simulink model "hw_sodim"  (R2017b)
settings: Solver=VariableStepAuto  StartTime=0.0  StopTime=inf  RelTol=1e-3  EnableMultiTasking=on
undefined symbols (not defined in the file or in its folder): A, N
libraries: xbsIndex_r4 x1, JTAGRuntimeCosim_r4 x1
settings Model: Creator=szekelyi  LastModifiedBy=kovacs.attila
settings DataIOCC: LimitDataPoints=on
settings OptimizationCC: LifeSpan=inf
settings DebuggingCC: AllowSymbolicDim=off  SFUnexpectedBacktrackingDiag=warning  SFNoUnconditionalDefaultTransitionDiag=warning  SFExecutionAtInitializationDiag=none
settings ModelReferenceCC: PropagateSignalLabelsOutOfModel=off
settings CodeAppCC: StateflowObjectComments=on
settings GRTTargetCC: TargetLangStandard=C89/C90 (ANSI)
settings ConfigComp: CovMetricSettings=dw  CovHtmlReporting=on  CovSaveCumulativeToWorkspaceVar=on  CovSaveSingleToWorkspaceVar=on  CovExternalEMLEnable=off

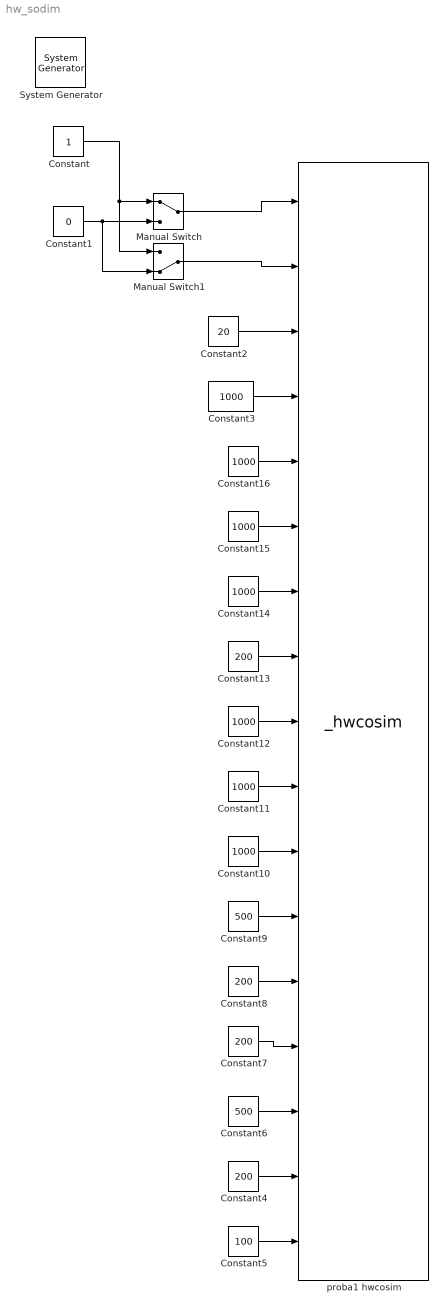
== system hw_sodim ==
  " System Generator" : xbsIndex_r4/ System Generator  Tag=genX  xilinxfamily=artix7  part=xc7a200t  speed=-2  package=fbg676  synthesis_tool=Vivado  clock_wrapper=Clock Enables  directory=./netlist  proj_type=Vivado  Synth_file=Vivado Synthesis Defaults  Impl_file=Vivado Implementation Defaults  testbench=off  simulink_period=1  sysclk_period=10  dcm_input_clock_period=10  incr_netlist=off  trim_vbits=Everywhere in SubSystem  dbl_ovrd=According to Block Masks  core_generation=According to Block Masks  run_coregen=off  deprecated_control=off  eval_field=0  block_type=sysgen
  Constant : Constant
  Constant1 : Constant  Value=0
  Constant{3,10..12,14..16} (7 alike) : Constant  Value=1000
  Constant{4,7..8,13} (4 alike) : Constant  Value=200
  Constant2 : Constant  Value=20
  Constant5 : Constant  Value=100
  Constant6 : Constant  Value=500
  Constant9 : Constant  Value=500
  Manual Switch : ManualSwitch
  Manual Switch1 : ManualSwitch  CurrentSetting=0
  proba1 hwcosim : JTAGRuntimeCosim_r4/_hwcosim  clkSrc=Single Stepped  hasCombinationalPath=on  bitfileName=D:\Diak\Kovacs_Attila\Demo\netlist\proba1.bit  skipConfig=off  dispPartInfo=off  useZynqReconfigScript=on  cable=Auto Detect  speed=N/A  cablePort=N/A  cableLocation=Local  shareCable=off  design_xtable=|  engineDll=JTAGCosimEngine.dll  cableWaitTime=10  bscanPos=-1  IRLengths=[]  useWaitBox=1  hasBufgmux=on  Scheme=Cosim  useCmdProc=1  hasProc=0  useImpact=0  printLogFile=0  userChain=2  block_type=jtagcosim
      | {
      |     'clkWrapper' => 'proba1',
      |     'burstMode' => false,
      |     'burstFifoDepth' => '1024',
      |     'shared_memories' => {},
      |     'clocksGcd' => 1,
      |     'device' => {
      |       'family' => 'artix7',
      |       'part' => 'xc7a35t',
      |       'package' => 'cpg236',
      |       'speed' => '-1',
      |     },
      |     'ports' => {
      |       'start' => {
      |         'direction' => 'in',
      |         'width' => 1,
      |         'name' => 'start',
      |         'period' => 1,
      |         'icon_text' => 'start',
      |         'type' => 'Bool',
      |         'arithmetic_type' => 'xlUnsigned',
      |         'dat_file' => 'proba1_jtag_domain_start.dat',
      |         'bin_pt' => 0,
      |         'addr_offset' => 0,
      |         'bd_port_index' => 0,
      |       },
      |       'reset' => {
      |         'direction' => 'in',
      |         'width' => 1,
      |         'name' => 'reset',
      |         'period' => 1,
      |         'icon_text' => 'reset',
      |         'type' => 'Bool',
      |         'arithmetic_type' => 'xlUnsigned',
      |         'dat_file' => 'proba1_jtag_domain_reset.dat',
      |         'bin_pt' => 0,
      |         'addr_offset' => 4,
      |         'bd_port_index' => 1,
      |       },
      |       'minval' => {
      |         'direction' => 'in',
      |         'width' => 32,
      |         'name' => 'minval',
      |         'period' => 1,
      |         'icon_text' => 'minval',
      |         'type' => 'UFix_32_0',
      |         'arithmetic_type' => 'xlUnsigned',
      |         'dat_file' => 'proba1_jtag_domain_minval.dat',
      |         'bin_pt' => 0,
      |         'addr_offset' => 8,
      |         'bd_port_index' => 2,
      |       },
      |       'maxval' => {
      |         'direction' => 'in',
      |         'width' => 32,
      |         'name' => 'maxval',
      |         'period' => 1,
      |         'icon_text' => 'maxval',
      |         'type' => 'UFix_32_0',
      |         'arithmetic_type' => 'xlUnsigned',
      |         'dat_file' => 'proba1_jtag_domain_maxval.dat',
      |         'bin_pt' => 0,
      |         'addr_offset' => 12,
      |         'bd_port_index' => 3,
      |       },
      |       'h9' => {
      |         'direction' => 'in',
      |         'width' => 32,
      |         'name' => 'h9',
      |         'period' => 1,
      |         'icon_text' => 'h9',
      |         'type' => 'UFix_32_0',
      |         'arithmetic_type' => 'xlUnsigned',
      |         'dat_file' => 'proba1_jtag_domain_h9.dat',
      |         'bin_pt' => 0,
      |         'addr_offset' => 16,
      |         'bd_port_index' => 4,
      |       },
      |       'h8' => {
      |         'direction' => 'in',
      |         'width' => 32,
      |         'name' => 'h8',
      |         'period' => 1,
      |         'icon_text' => 'h8',
      |         'type' => 'UFix_32_0',
      |         'arithmetic_type' => 'xlUnsigned',
      |         'dat_file' => 'proba1_jtag_domain_h8.dat',
      |         'bin_pt' => 0,
      |         'addr_offset' => 20,
      |         'bd_port_index' => 5,
      |       },
      |       'h7' => {
      |         'direction' => 'in',
      |         'width' => 32,
      |         'name' => 'h7',
      |         'period' => 1,
      |         'icon_text' => 'h7',
      |         'type' => 'UFix_32_0',
      |         'arithmetic_type' => 'xlUnsigned',
      |         'dat_file' => 'proba1_jtag_domain_h7.dat',
      |         'bin_pt' => 0,
      |         'addr_offset' => 24,
      |         'bd_port_index' => 6,
      |       },
      |       'h6' => {
      |         'direction' => 'in',
      |         'width' => 32,
      |         'name' => 'h6',
      |         'period' => 1,
      |         'icon_text' => 'h6',
      |         'type' => 'UFix_32_0',
      |         'arithmetic_type' => 'xlUnsigned',
      |         'dat_file' => 'proba1_jtag_domain_h6.dat',
      |         'bin_pt' => 0,
      |         'addr_offset' => 28,
      |         'bd_port_index' => 7,
      |       },
      |       'h5' => {
      |         'direction' => 'in',
      |         'width' => 32,
      |         'name' => 'h5',
      |         'period' => 1,
      |         'icon_text' => 'h5',
      |         'type' => 'UFix_32_0',
      |         'arithmetic_type' => 'xlUnsigned',
      |         'dat_file' => 'proba1_jtag_domain_h5.dat',
      |         'bin_pt' => 0,
      |         'addr_offset' => 32,
      |         'bd_port_index' => 8,
      |       },
      |       'h4' => {
      |         'direction' => 'in',
      |         'width' => 32,
      |         'name' => 'h4',
      |         'period' => 1,
      |         'icon_text' => 'h4',
      |         'type' => 'UFix_32_0',
      |         'arithmetic_type' => 'xlUnsigned',
      |         'dat_file' => 'proba1_jtag_domain_h4.dat',
      |         'bin_pt' => 0,
      |         'addr_offset' => 36,
      |         'bd_port_index' => 9,
      |       },
      |       'h3' => {
      |         'direction' => 'in',
      |         'width' => 32,
      |         'name' => 'h3',
      |         'period' => 1,
      |         'icon_text' => 'h3',
      |         'type' => 'UFix_32_0',
      |         'arithmetic_type' => 'xlUnsigned',
      |         'dat_file' => 'proba1_jtag_domain_h3.dat',
      |         'bin_pt' => 0,
      |         'addr_offset' => 40,
      |         'bd_port_index' => 10,
      |       },
      |       'h2' => {
      |         'direction' => 'in',
      |         'width' => 32,
      |         'name' => 'h2',
      |         'period' => 1,
      |         'icon_text' => 'h2',
      |         'type' => 'UFix_32_0',
      |         'arithmetic_type' => 'xlUnsigned',
      |         'dat_file' => 'proba1_jtag_domain_h2.dat',
      |         'bin_pt' => 0,
      |         'addr_offset' => 44,
      |         'bd_port_index' => 11,
      |       },
      |       'h11' => {
      |         'direction' => 'in',
      |         'width' => 32,
      |         'name' => 'h11',
      |         'period' => 1,
      |         'icon_text' => 'h11',
      |         'type' => 'UFix_32_0',
      |         'arithmetic_type' => 'xlUnsigned',
      |         'dat_file' => 'proba1_jtag_domain_h11.dat',
      |         'bin_pt' => 0,
      |         'addr_offset' => 48,
      |         'bd_port_index' => 12,
      |       },
      |       'h10' => {
      |         'direction' => 'in',
      |         'width' => 32,
      |         'name' => 'h10',
      |         'period' => 1,
      |         'icon_text' => 'h10',
      |         'type' => 'UFix_32_0',
      |         'arithmetic_type' => 'xlUnsigned',
      |         'dat_file' => 'proba1_jtag_domain_h10.dat',
      |         'bin_pt' => 0,
      |         'addr_offset' => 52,
      |         'bd_port_index' => 13,
      |       },
      |       'h1' => {
      |         'direction' => 'in',
      |         'width' => 32,
      |         'name' => 'h1',
      |         'period' => 1,
      |         'icon_text' => 'h1',
      |         'type' => 'UFix_32_0',
      |         'arithmetic_type' => 'xlUnsigned',
      |         'dat_file' => 'proba1_jtag_domain_h1.dat',
      |         'bin_pt' => 0,
      |         'addr_offset' => 56,
      |         'bd_port_index' => 14,
      |       },
      |       'h' => {
      |         'direction' => 'in',
      |         'width' => 32,
      |         'name' => 'h',
      |         'period' => 1,
      |         'icon_text' => 'h',
      |         'type' => 'UFix_32_0',
      |         'arithmetic_type' => 'xlUnsigned',
      |         'dat_file' => 'proba1_jtag_domain_h.dat',
      |         'bin_pt' => 0,
      |         'addr_offset' => 60,
      |         'bd_port_index' => 15,
      |       },
      |       'divval' => {
      |         'direction' => 'in',
      |         'width' => 10,
      |         'name' => 'divval',
      |         'period' => 1,
      |         'icon_text' => 'divval',
      |         'type' => 'UFix_10_0',
      |         'arithmetic_type' => 'xlUnsigned',
      |         'dat_file' => 'proba1_jtag_domain_divval.dat',
      |         'bin_pt' => 0,
      |         'addr_offset' => 64,
      |         'bd_port_index' => 16,
      |       },
      |     },
      |   }
  wires:
  Constant/1 -> Manual Switch1/1, Manual Switch/1
  Constant1/1 -> Manual Switch1/2, Manual Switch/2
  Manual Switch/1 -> proba1 hwcosim/1
  Manual Switch1/1 -> proba1 hwcosim/2
  Constant2/1 -> proba1 hwcosim/3
  Constant3/1 -> proba1 hwcosim/4
  Constant4/1 -> proba1 hwcosim/16
  Constant5/1 -> proba1 hwcosim/17
  Constant16/1 -> proba1 hwcosim/5
  Constant15/1 -> proba1 hwcosim/6
  Constant14/1 -> proba1 hwcosim/7
  Constant13/1 -> proba1 hwcosim/8
  Constant12/1 -> proba1 hwcosim/9
  Constant11/1 -> proba1 hwcosim/10
  Constant10/1 -> proba1 hwcosim/11
  Constant9/1 -> proba1 hwcosim/12
  Constant8/1 -> proba1 hwcosim/13
  Constant7/1 -> proba1 hwcosim/14
  Constant6/1 -> proba1 hwcosim/15
